simulink model "ext_mode_intro"  (R2017b)
settings: Solver=FixedStepDiscrete  StartTime=0.0  StopTime=inf  RelTol=1e-3  EnableMultiTasking=on
InitFcn:
  | GainTune = 1;
libraries: pixhawk_slib_sensors_actuators x1
Description:
  | ext_mode_intro
  | 
  | This model uses ttyS6 on the Pixhawk for the EXT mode serial data exchange.
  | This means the MEX arguments must be set accordingly to use the right COM port.
  | Please check your windows setting (COM8 in this example)
  | COM 6 will be the serial console (ttyACM0)
  | 
  | Note: Baud rate set at 115200
settings Model: SimulationMode=external  Creator=skuznick  LastModifiedBy=skuznick
settings DataIOCC: LimitDataPoints=on  SaveFormat=Array  SignalLoggingSaveFormat=ModelDataLogs
settings OptimizationCC: DefaultParameterBehavior=Inlined  LifeSpan=1  MaxStackSize=64
settings DebuggingCC: SolverPrmCheckMsg=warning  MultiTaskDSMMsg=warning  MultiTaskCondExecSysMsg=none  AllowSymbolicDim=off  SFUnexpectedBacktrackingDiag=warning  SFNoUnconditionalDefaultTransitionDiag=warning  SFExecutionAtInitializationDiag=none
settings HardwareCC: ProdBitPerPointer=32  ProdBitPerSizeT=32  ProdBitPerPtrDiffT=32  ProdLargestAtomicInteger=Long  ProdLargestAtomicFloat=Double  ProdIntDivRoundTo=Undefined  ProdWordSize=32  ProdHWDeviceType=ARM Compatible->ARM Cortex
settings ModelReferenceCC: PropagateSignalLabelsOutOfModel=off
settings SFSimCC: MATLABDynamicMemAlloc=off
settings RTWCC: SystemTargetFile=ert.tlc  HardwareBoard=Pixhawk PX4  TLCOptions=-aInlineSetEventsForThisBaseRateFcn=TLC_FALSE -aSuppressMultiTaskScheduler=TLC_FALSE -aRateBasedStepFcn=0  TemplateMakefile=ert_default_tmf  GenerateReport=on  Toolchain=Pixhawk Toolchain  IncludeHyperlinkInReport=on  LaunchReport=on  GenerateTraceInfo=on  GenerateTraceReport=on  GenerateTraceReportSl=on  GenerateTraceReportSf=on  GenerateTraceReportEml=on  GenerateCodeMetricsReport=on
settings CodeAppCC: IgnoreCustomStorageClasses=off  StateflowObjectComments=on
settings ERTTargetCC: MultiwordLength=2048  ExtMode=on  ExtModeTransport=1  ExtModeStaticAllocSize=10000  ExtModeMexFile=ext_serial_win32_comm  ExtModeMexArgs=1 8 115200 5  ERTCustomFileTemplate=px4_codertarget_file_process.tlc  ConvertIfToSwitch=off  SuppressUnreachableDefaultCases=off
settings ConfigComp: CovMetricSettings=dw  CovHtmlReporting=on  CovSaveCumulativeToWorkspaceVar=on  CovSaveSingleToWorkspaceVar=on  CovExternalEMLEnable=off  CovSFcnEnable=off

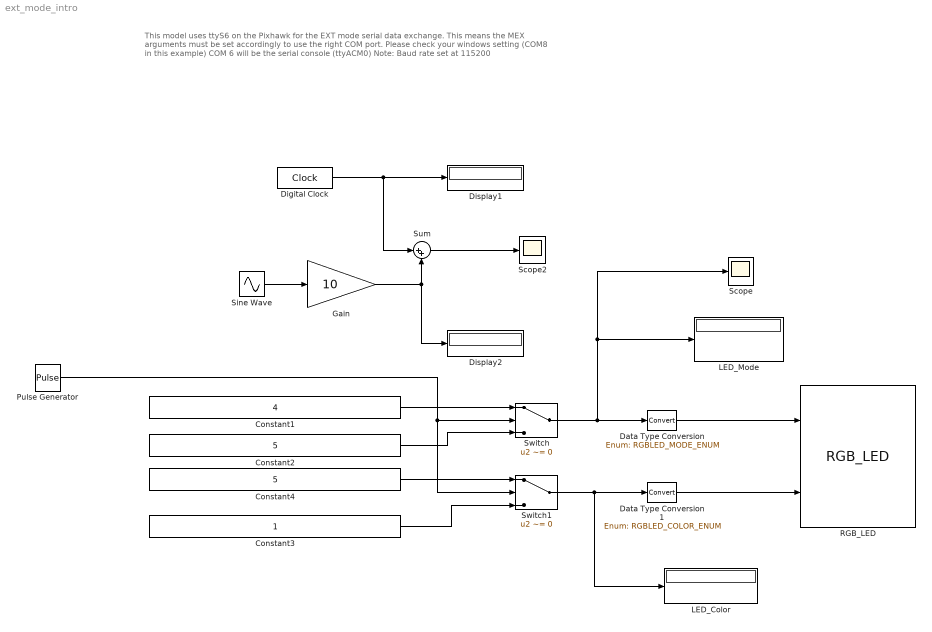
== system ext_mode_intro ==
  note: This model uses ttyS6 on the Pixhawk for the EXT mode serial data exchange.
      | This means the MEX arguments must be set accordingly to use the right COM port.
      | Please check your windows setting (COM8 in this example)
      | COM 6 will be the serial console (ttyACM0)
      |
      | Note: Baud rate set at 115200
  Constant1 : Constant  Value=4  OutDataTypeStr=int8
  Constant2 : Constant  Value=5  OutDataTypeStr=int8
  Constant3 : Constant  OutDataTypeStr=int8
  Constant4 : Constant  Value=5  OutDataTypeStr=int8
  Data Type Conversion : DataTypeConversion  OutDataTypeStr=Enum: RGBLED_MODE_ENUM
  Data Type Conversion1 : DataTypeConversion  OutDataTypeStr=Enum: RGBLED_COLOR_ENUM
  Digital Clock : DigitalClock  SampleTime=0.1
  Display1 : Display
  Display2 : Display
  Gain : Gain  Gain=10
  LED_Color : Display
  LED_Mode : Display
  Pulse Generator : DiscretePulseGenerator  PulseType=Time based  Period=6  PulseWidth=50
  RGB_LED : pixhawk_slib_sensors_actuators/RGB_LED
      settings: SourceProductName=Pixhawk Target Blocks
  Scope : Scope
  Scope2 : Scope
  Sine Wave : Sin  SampleTime=0.1
  Sum : Sum  Inputs=|++
  Switch : Switch  Criteria=u2 ~= 0  Threshold=1500
  Switch1 : Switch  Criteria=u2 ~= 0  Threshold=1500
  wires:
  Switch/1 -> Scope/1, LED_Mode/1, Data Type Conversion/1
  Switch1/1 -> LED_Color/1, Data Type Conversion1/1
  Constant1/1 -> Switch/1
  Constant2/1 -> Switch/3
  Constant4/1 -> Switch1/1
  Constant3/1 -> Switch1/3
  Pulse Generator/1 -> Switch1/2, Switch/2
  Digital Clock/1 -> Sum/1, Display1/1
  Data Type Conversion/1 -> RGB_LED/1
  Data Type Conversion1/1 -> RGB_LED/2
  Sine Wave/1 -> Gain/1
  Sum/1 -> Scope2/1
  Gain/1 -> Sum/2, Display2/1
